simulink model "terminal_sliding_mode"  (R2019b)
settings: Solver=VariableStepAuto  StartTime=0.0  StopTime=10  RelTol=1e-3
settings Model: Creator=Alien  LastModifiedBy=Alien

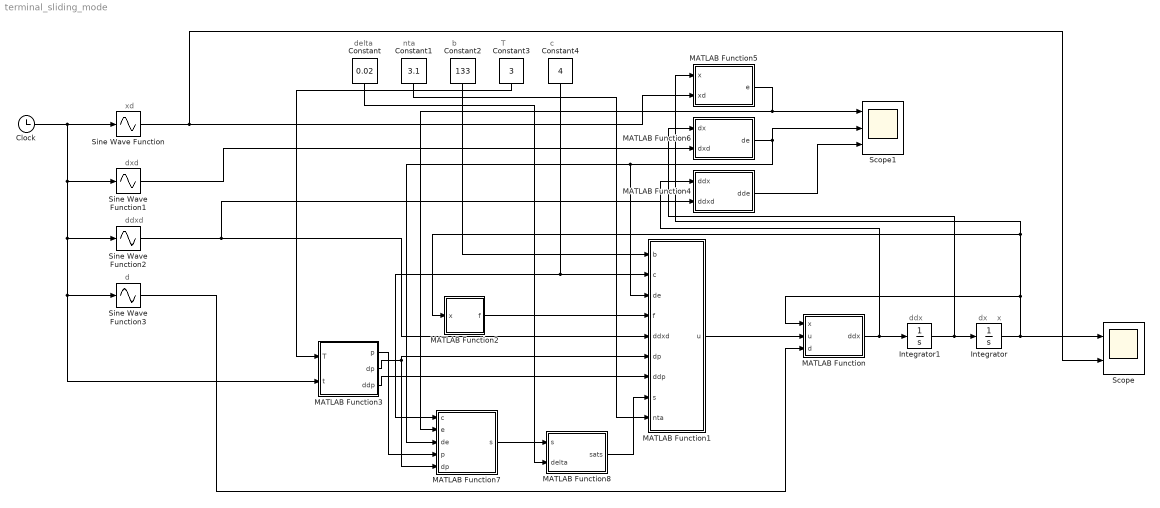
== system terminal_sliding_mode ==
  note: xd
  note: ddx
  note: dx
  note: x
  note: nta
  note: delta
  note: T
  note: b
  note: c
  note: dxd
  note: ddxd
  note: d
  Clock : Clock
  Constant : Constant  Value=0.02
  Constant1 : Constant  Value=3.1
  Constant2 : Constant  Value=133
  Constant3 : Constant  Value=3
  Constant4 : Constant  Value=4
  Integrator : Integrator
  Integrator1 : Integrator  InitialCondition=0.5
  MATLAB Function : MATLAB Function  TreatAsAtomicUnit=on
  MATLAB Function1 : MATLAB Function  TreatAsAtomicUnit=on
  MATLAB Function2 : MATLAB Function  TreatAsAtomicUnit=on
  MATLAB Function3 : MATLAB Function  TreatAsAtomicUnit=on
  MATLAB Function4 : MATLAB Function  TreatAsAtomicUnit=on
  MATLAB Function5 : MATLAB Function  TreatAsAtomicUnit=on
  MATLAB Function6 : MATLAB Function  TreatAsAtomicUnit=on
  MATLAB Function7 : MATLAB Function  TreatAsAtomicUnit=on
  MATLAB Function8 : MATLAB Function  TreatAsAtomicUnit=on
  Scope : Scope  NumInputPorts=2
  Scope1 : Scope  NumInputPorts=3
  Sine Wave Function : Sin  TimeSource=Use external signal  SampleTime=0
  Sine Wave Function1 : Sin  TimeSource=Use external signal  Phase=pi/2  SampleTime=0
  Sine Wave Function2 : Sin  TimeSource=Use external signal  Amplitude=-1  SampleTime=0
  Sine Wave Function3 : Sin  TimeSource=Use external signal  Amplitude=3  Frequency=2*pi  SampleTime=0
  wires:
  Integrator1/1 -> MATLAB Function6/1(dx), Integrator/1
  MATLAB Function/1(ddx) -> MATLAB Function4/1(ddx), Integrator1/1
  MATLAB Function1/1(u) -> MATLAB Function/2(u)
  MATLAB Function2/1(f) -> MATLAB Function1/4(f)
  Integrator/1 -> Scope/1, MATLAB Function2/1(x), MATLAB Function5/1(x), MATLAB Function/1(x)
  MATLAB Function8/1(sats) -> MATLAB Function1/8(s)
  MATLAB Function7/1(s) -> MATLAB Function8/1(s)
  MATLAB Function3/1(p) -> MATLAB Function7/4(p)
  MATLAB Function3/2(dp) -> MATLAB Function1/6(dp), MATLAB Function7/5(dp)
  MATLAB Function3/3(ddp) -> MATLAB Function1/7(ddp)
  MATLAB Function6/1(de) -> Scope1/2, MATLAB Function7/3(de), MATLAB Function1/3(de)
  MATLAB Function5/1(e) -> Scope1/1, MATLAB Function7/2(e)
  Constant1/1 -> MATLAB Function1/9(nta)
  Constant/1 -> MATLAB Function8/2(delta)
  Constant4/1 -> MATLAB Function7/1(c), MATLAB Function1/2(c)
  Constant2/1 -> MATLAB Function1/1(b)
  Clock/1 -> MATLAB Function3/2(t), Sine Wave Function3/1, Sine Wave Function2/1, Sine Wave Function1/1, Sine Wave Function/1
  Sine Wave Function/1 -> Scope/2, MATLAB Function5/2(xd)
  Sine Wave Function1/1 -> MATLAB Function6/2(dxd)
  Sine Wave Function2/1 -> MATLAB Function1/5(ddxd), MATLAB Function4/2(ddxd)
  Sine Wave Function3/1 -> MATLAB Function/3(d)
  Constant3/1 -> MATLAB Function3/1(T)
  MATLAB Function4/1(dde) -> Scope1/3

== matlab function terminal_sliding_mode/MATLAB Function1 ==
  data: b input; u output; c input; de input; f input; ddxd input; dp input; ddp input; s input; nta input
function u = fcn(b, c, de, f, ddxd, dp, ddp, s, nta)
u = -1/b*(1/c*(de - dp) + f - ddxd - ddp + nta*s);

== matlab function terminal_sliding_mode/MATLAB Function ==
  data: x input; u input; ddx output; d input
function ddx = fcn(x, u, d)
ddx = -25 * x + 133 * u + d;

== matlab function terminal_sliding_mode/MATLAB Function2 ==
  data: x input; f output
function f = fcn(x)
f = -25 * x;

== matlab function terminal_sliding_mode/MATLAB Function3 ==
  settings: updateMethod=DISCRETE
  data: T input; p output; t input; dp output; ddp output
function [p, dp, ddp] = fcn(T, t)
persistent A1 A2 A3 e0 de0 dde0;

if isempty(A1)
%     A1 = 0;A2 = 0;A3 = 0;
    e0 = 0;de0 = -0.5; dde0 = 6.3;
    A1 = 10/T^3 * e0 + 6/T^2 * de0 + 3/(2 * T) * dde0;
    A2 = 15/T^4 * e0 + 8/T^3 * de0 + 3/(2 * T^2) * dde0;
    A3 = 6/T^5 * e0 + 3/T^4 * de0 + 1/(2 * T^3) * dde0;
end
% if(t==1)
%     A1 = 10/T^3 * e0 + 6/T^2 * de0 + 3/(2 * T) * dde0;
%     A2 = 15/T^4 * e0 + 8/T^3 * de0 + 3/(2 * T^2) * dde0;
%     A3 = 6/T^5 * e0 + 3/T^4 * de0 + 3/(2 * T^3) * dde0;
% end

if(t<=T)
    p = e0 + de0 * t + 0.5 * dde0 * t^2 - A1 * t^3 + A2 * t^4 - A3 * t^5;
    dp = de0 + dde0 * t - 3 * A1 * t^2 + 4 * A2 * t^3 - 5 * A3 * t^4;
    ddp = dde0 - 6 * A1 * t + 12 * A2 * t^2 - 20 * A3 * t^3;
else
    p = 0;dp = 0; ddp = 0;
end

== matlab function terminal_sliding_mode/MATLAB Function4 ==
  data: ddx input; dde output; ddxd input
function dde = fcn(ddx, ddxd)
dde = ddx - ddxd;

== matlab function terminal_sliding_mode/MATLAB Function5 ==
  data: x input; e output; xd input
function e = fcn(x, xd)
e = x - xd;

== matlab function terminal_sliding_mode/MATLAB Function6 ==
  data: dx input; de output; dxd input
function de = fcn(dx, dxd)
de = dx - dxd;

== matlab function terminal_sliding_mode/MATLAB Function7 ==
  data: c input; s output; e input; de input; p input; dp input
function s = fcn(c, e, de, p, dp)
s = (c * e + de) - (c * p + dp);

== matlab function terminal_sliding_mode/MATLAB Function8 ==
  data: s input; sats output; delta input
function sats = fcn(s, delta)
kk = 1/delta;
if(s > delta)
    sats = 1;
elseif(s < -delta)
    sats = -1;
else
    sats = kk * s;
end
